simulink model "LoadFlow58BusNetwork_2023"  (R2023b)
settings: Solver=FixedStepDiscrete  StartTime=0.0  StopTime=4.5  FixedStep=75e-6  RelTol=1e-3  EnableMultiTasking=on
undefined symbols (not defined in the file): D1, D11, Delta
libraries: spsSeriesRLCBranchLib x41, spsLoadFlowBusLib x29, spsDistributedParametersLineLib x19, spsThreePhaseSeriesRLCLoadLib x15, spsThreePhaseTransformerTwoWindingsLib x13, spsThreePhaseParallelRLCLoadLib x11, spsThreePhaseVIMeasurementLib x11, spsSynchronousMachinepuStandardLib x7, spsExcitationSystemLib x7, spsHydraulicTurbineandGovernorLib x7, spsGenericPowerSystemStabilizerLib x7, spsMultiBandPowerSystemStabilizerLib x7
(part 1 of 5)
settings Model: Creator=The MathWorks, Inc.  LastModifiedBy=dilu2
settings SolverCC: AlgebraicLoopSolver=TrustRegion
settings DataIOCC: SaveFormat=StructureWithTime  SaveOutput=off  SignalLogging=off  DSMLogging=off  SaveTime=off  ReturnWorkspaceOutputs=off
settings OptimizationCC: ExpressionDepthLimit=2147483647  LifeSpan=inf
settings DebuggingCC: UnderspecifiedInitializationDetection=Classic  MergeDetectMultiDrivingBlocksExec=none  SolverPrmCheckMsg=warning  FcnCallInpInsideContextMsg=warning  UnconnectedInputMsg=warning  UnconnectedOutputMsg=warning  UnconnectedLineMsg=warning  StateNameClashWarn=warning  SFUnexpectedBacktrackingDiag=warning  SFNoUnconditionalDefaultTransitionDiag=warning  SFExecutionAtInitializationDiag=none  ArithmeticOperatorsInVariantConditions=warning
settings HardwareCC: ProdBitPerPointer=32  ProdBitPerSizeT=32  ProdBitPerPtrDiffT=32  ProdLargestAtomicFloat=None  ProdIntDivRoundTo=Undefined  ProdEndianess=Unspecified  ProdWordSize=32  ProdHWDeviceType=32-bit Generic
settings ModelReferenceCC: EnableRefExpFcnMdlSchedulingChecks=on  PropagateSignalLabelsOutOfModel=off
settings SFSimCC: SimUseLocalCustomCode=off  CustomCodeUndefinedFunction=UseInterfaceOnly
settings RTWCC: RTWUseLocalCustomCode=off
settings CodeAppCC: StateflowObjectComments=on
settings GRTTargetCC: TargetLangStandard=C89/C90 (ANSI)  CombineOutputUpdateFcns=off  GRTInterface=on
settings ConfigComp: CovMetricSettings=dw  CovSaveCumulativeToWorkspaceVar=on  CovSaveSingleToWorkspaceVar=on  CovExternalEMLEnable=off  CovSFcnEnable=off
settings SimscapeCC: SimscapeNormalizeSystem=off

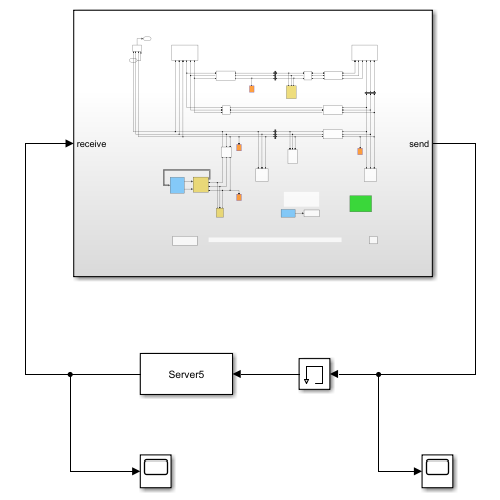
[thumbnail: Simulink's stored preview of the top-level diagram]
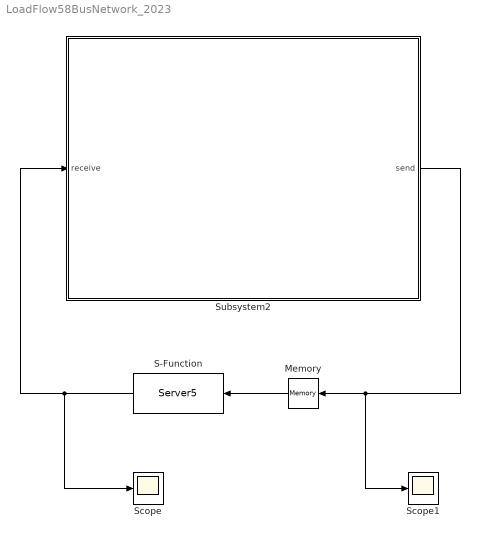
== system LoadFlow58BusNetwork_2023 ==
  Memory : Memory
  S-Function : S-Function  FunctionName=Server5  SFunctionDeploymentMode=off  EnableBusSupport=off
  Scope : Scope
  Scope1 : Scope
  Subsystem2 : Subsystem
  wires:
  Memory/1 -> S-Function/1
  Subsystem2/1(send) -> Scope1/1, Memory/1
  S-Function/1 -> Scope/1, Subsystem2/1(receive)

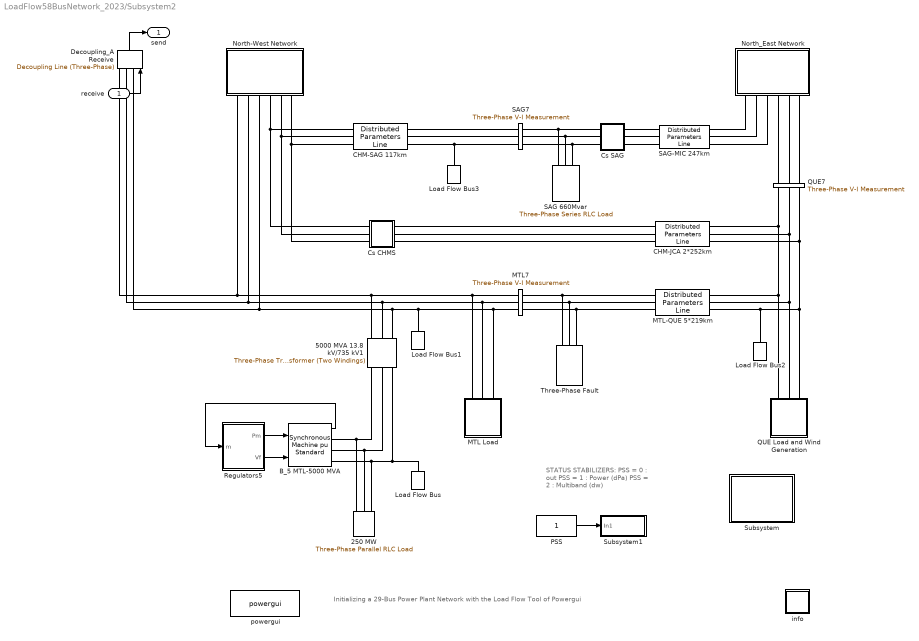
== system LoadFlow58BusNetwork_2023/Subsystem2 ==
  note: Initializing a 29-Bus Power Plant Network with the Load Flow Tool of Powergui
  note: STATUS STABILIZERS:
      | PSS = 0 :  out
      | PSS = 1 :  Power (dPa)
      | PSS = 2 :  Multiband (dw)
  receive : Inport
  250 MW : spsThreePhaseParallelRLCLoadLib/Three-Phase Parallel RLC Load  LConnTagsString=A|B|C  Configuration=Y (grounded)  NominalVoltage=(13800)*1  Vabc=[1e3 1e3 1e3]  Vabcp=[1e3 1e3 1e3]  NominalFrequency=60  UnbalancedPower=off  ActivePower=250000000  InductivePower=0  CapacitivePower=0  Pabc=[10e3 9e3 11e3]  QLabc=[100 90 110]  QCabc=[100 90 110]  Pabcp=[10e3 9e3 11e3]  QLabcp=[100 90 110]  QCabcp=[100 90 110]  Measurements=None  LoadType=constant PQ
  5000 MVA 13.8 kV/735 kV1 : spsThreePhaseTransformerTwoWindingsLib/Three-Phase Transformer (Two Windings)  Winding1Connection=Delta (D1)  Winding2Connection=Yg  CoreType=Three single-phase transformers  SetSaturation=off  Hysteresis=off  DataFile='basic_model'  SetInitialFlux=off  Measurements=None  UNITS=pu  NominalPower=[ 5000e6 60 ]  Winding1="[ 13.8e3 0.002  0.0]"  Winding2=[ 735e3 0.002 0.12]  Rm=500  Lm=500  L0=0.5  Saturation="[ 0,0  ;  0.005,1.2  ;  1.0,1.4 ]"  InitialFluxes=[ 0.8 , -0.8 , 0.7 ]  BreakLoop=off  DiscreteSolver=Trapezoidal iterative  DataType=off  TransfoNumber=0
  B_5 MTL-5000 MVA : spsSynchronousMachinepuStandardLib/Synchronous Machine pu Standard  PresetModel=No  MechanicalLoad=Mechanical power Pm  ShowDetailedParameters=on  RotorType=Salient-pole  Units=per unit standard parameters  MeasurementBus=off  NominalParameters="[5000E6  13800   60 ]"  Reactances1=[ 31 32 33 34 35 36 37 ]  Reactances2=[ 1.305, 0.296, 0.252, 0.474, 0.243, 0.18 ]  dAxisTimeConstants=Short-circuit  qAxisTimeConstants=Open-circuit  TimeConstants1=[]  TimeConstants2=[]  TimeConstants3=[]  TimeConstants4=[]  TimeConstants5=[ 1.01, 0.053, 0.1 ]  TimeConstants6=[]  TimeConstants7=[]  TimeConstants8=[]  StatorResistance=2.8544e-3  Mechanical="[ 3.7 0  32]"  PolePairs=32  InitialConditions=[0 -113.876 0.904539 0.904539 0.904539 -42.1129 -162.113 77.8871 1.28555]  SetSaturation=off  Saturation=[0.6404,0.7127,0.8441,0.9214,0.9956,1.082,1.19,1.316,1.457;0.7,0.7698,0.8872,0.9466,0.9969,1.046,1.1,1.151,1.201]  LoadFlowParameters=[1 4000000000 0 0 0]  TsPowergui=0  TsBlock=-1  IterativeModel=Trapezoidal non iterative  IterativeDiscreteModel=Trapezoidal non iterative  BusType=PV  Pref=4500000000  Qref=0  Qmin=-Inf  Qmax=Inf  PLF=0  QLF=0
  CHM-JCA 2*252km : spsDistributedParametersLineLib/Distributed Parameters Line  Phases=3  Length=252  Frequency=60  Resistance="[0.01273  0.3864]/2"  Inductance="[0.9337e-3  4.1264e-3]/2"  Capacitance=[12.74e-9 7.751e-9]*2  x1=[-0.0015 2.03674165345122e-08 15714.2625948716 -742648.807936692;-0.001425 2.03855691202494e-08 36703.0761534828 -741907.711972198;-0.00135 2.03874257939416e-08 57662.5498345927 -740573.546334321;-0.001275 2.03729850713921e-08 78575.9289556316 -738647.377534661;-0.0012 2.03422584962937e-08 99426.4956813152 -736130.745323082;-0.001125 2.02952706310004e-08 120197.582387628 -733025.661456871;-0.00105 2.02320590368927e-08 140872.584985664 -729334.60809256;-0.000975 2.01526742443518e-08 161434.976194686 -725060.535801733;-0.0009 2.00571797123662e-08 181868.318753776 -720206.861212384;-0.000825 1.99456517778037e-08 202156.278561532 -714777.464277717;-0.00075 1.98181795943887e-08 222282.637733301 -708776.685174569;-0.000675 1.96748650614343e-08 242231.307565505 -702209.320833938;-0.0006 1.95158227423853e-08 261986.341396704 -695080.621106396;-0.000525 1.93411797732382e-08 281531.947355116 -687396.284565432;-0.00045 1.91510757609102e-08 300852.500982395 -679162.453952101;-0.000375 1.89456626716403e-08 319932.557723587 -670385.711264616;-0.0003 1.87251047095091e-08 338756.865273267 -661073.072496791;-0.000225 1.84895781851768e-08 357310.375768001 -651231.982029569;-0.00015 1.82392713749432e-08 375578.257815379 -640870.306680096;-7.5e-05 1.79743843702428e-08 393545.908349999 -629996.329413108]  x2=[-0.0015 1.37869966912524e-08 -209700.60363331 -700128.672634898;-0.001425 1.37569590076229e-08 -189823.746323567 -705777.19657371;-0.00135 1.37159242214512e-08 -169795.146815414 -710861.533020335;-0.001275 1.36639251353176e-08 -149630.815664849 -715377.617634008;-0.0012 1.36010033164958e-08 -129346.87192967 -719321.84032579;-0.001125 1.35272090637252e-08 -108959.530284144 -722691.048144409;-0.00105 1.34426013670023e-08 -88485.0880572453 -725482.547796685;-0.000975 1.33472478604253e-08 -67939.9122048211 -727694.107800508;-0.0009 1.32412247681284e-08 -47340.4262260959 -729323.960268648;-0.000825 1.31246168433494e-08 -26703.0970349784 -730370.80232198;-0.00075 1.29975173006792e-08 -6044.42179666215 -730833.797130983;-0.000675 1.28600277415475e-08 14619.0852599556 -730712.574584693;-0.0006 1.27122580730043e-08 35270.906043496 -730007.231586556;-0.000525 1.25543264198615e-08 55894.5318044082 -728718.331976975;-0.00045 1.23863590302664e-08 76473.476331811 -726846.906082576;-0.000375 1.22084901747801e-08 96991.2891323175 -724394.449892584;-0.0003 1.20208620390443e-08 117431.568580308 -721362.923862956;-0.000225 1.18236246101198e-08 137777.975029139 -717754.751349214;-0.00015 1.16169355565895e-08 158014.243872805 -713572.81666926;-7.5e-05 1.14009601025203e-08 178124.198547619 -708820.46279769]  x3=[-0.0015 5.07994553465233e-11 0.894999888144781 -284.908126310178;-0.001425 5.0283598192617e-11 8.94952227203379 -284.768519995358;-0.00135 4.97275450996804e-11 16.9968905447508 -284.401274082759;-0.001275 4.91317405680481e-11 25.0306717632275 -283.806682143142;-0.0012 4.84966608747465e-11 33.0444438456788 -282.985219484209;-0.001125 4.78228136927654e-11 41.0318007053168 -281.937542770639;-0.00105 4.71107376852319e-11 48.9863573712786 -280.664489499167;-0.000975 4.63610020748113e-11 56.9017550926742 -279.1670773291;-0.0009 4.55742061886792e-11 64.7716664216747 -277.446503268816;-0.000825 4.47509789794286e-11 72.5898002715775 -275.504142718892;-0.00075 4.38919785222948e-11 80.3499069458043 -273.341548372634;-0.000675 4.29978914891001e-11 88.0457831338135 -270.960448974872;-0.0006 4.20694325993388e-11 95.6712768699312 -268.362747940034;-0.000525 4.11073440488415e-11 103.220292451139 -265.550521830581;-0.00045 4.0112394916475e-11 110.686795309884 -262.526018697035;-0.000375 3.90853805493524e-11 118.064816838024 -259.291656280926;-0.0003 3.80271219270451e-11 125.348459158035 -255.850020082081;-0.000225 3.69384650053039e-11 132.531899837691 -252.203861291819;-0.00015 3.58202800398148e-11 139.609396544424 -248.356094593689;-7.5e-05 3.46734608905305e-11 146.575291635653 -244.309795833516]  x4=[-0.0015 3.66725542612014e-11 -3172.83341993509 -10043.3125795462;-0.001425 3.78072265237595e-11 -2887.63550825212 -10128.9965094921;-0.00135 3.89116762679046e-11 -2600.12926492615 -10206.5834746072;-0.001275 3.99850206134097e-11 -2310.54451804911 -10276.0114530587;-0.0012 4.10264015452278e-11 -2019.11275723686 -10337.2249451828;-0.001125 4.20349865993756e-11 -1726.06694857993 -10390.1750178506;-0.00105 4.30099695283927e-11 -1431.64134841402 -10434.8193435841;-0.000975 4.39505709458435e-11 -1136.07131605904 -10471.1222343925;-0.0009 4.48560389493464e-11 -839.593125676469 -10499.0546703002;-0.000825 4.57256497216336e-11 -542.443777395441 -10518.5943225455;-0.00075 4.65587081091593e-11 -244.860807858432 -10529.7255714291;-0.000675 4.73545481777946e-11 52.9178996618857 -10532.4395188012;-0.0006 4.81125337451655e-11 350.654305422883 -10526.7339951737;-0.000525 4.88320588892069e-11 648.110403497316 -10512.6135614548;-0.00045 4.95125484325279e-11 945.048412031615 -10490.0895053033;-0.000375 5.01534584021993e-11 1241.23096332506 -10459.1798321051;-0.0003 5.07542764645976e-11 1536.4212935779 -10419.9092505798;-0.000225 5.13145223349566e-11 1830.38343215668 -10372.3091530296;-0.00015 5.18337481612995e-11 2122.8823902256 -10316.4175902441;-7.5e-05 5.23115388824452e-11 2413.68434859297 -10252.2792410835]  x5=0.00142516474882927  V1=ones(3,3)  V2=ones(3,3)  I1=ones(3,3)  I2=ones(3,3)  nHarmo=1  Measurements=None  Decoupling=on  VsMag0=[606505.937088283 606505.596193745 606505.952336163]  VrMag0=[596743.737336247 596743.91108333 596743.706580376]  VsAngle0=[3.61218308622859 -116.387796657598 123.612221103652]  VrAngle0=[-14.273856882172 -134.273869923449 105.726122150014]  IsMag0=[234.023435045969 234.01262310868 234.010085805348]  IrMag0=[8650.90032066037 8650.90619032997 8650.91364627855]  IsAngle0=[2.58186505622523 -117.420380634301 122.583034804805]  IrAngle0=[-15.1321830152103 -135.132103549667 104.867823050534]
      settings: AttributesFormatString=\n  LibrarySourceBlock=sps_lib/Power Grid Elements/Distributed Parameters Line
  CHM-SAG 117km : spsDistributedParametersLineLib/Distributed Parameters Line  Phases=3  Length=117  Frequency=60  Resistance="[0.01273  0.3864]"  Inductance="[0.9337e-3  4.1264e-3]"  Capacitance=[12.74e-9 7.751e-9]  x1=[-0.000675 1.89233254598605e-08 161384.253868475 -730188.013921104;-0.0006 1.87743600273455e-08 181962.578167373 -725333.731757204;-0.000525 1.86103866586821e-08 202395.444365406 -719899.628906115;-0.00045 1.84315364316721e-08 222666.518741967 -713890.049306513;-0.000375 1.82379523164507e-08 242759.596910358 -707309.796924379;-0.0003 1.80297890611975e-08 262658.616771325 -700164.131912787;-0.000225 1.78072130684338e-08 282347.671352857 -692458.766407013;-0.00015 1.75704022620027e-08 301811.021525973 -684199.859958349;-7.5e-05 1.73195459448395e-08 321033.108586345 -675394.014610243]  x2=[-0.000675 1.29805140179051e-08 211241.020698715 -709610.354234726;-0.0006 1.28522856813478e-08 231217.678579191 -703354.83438148;-0.000525 1.27137834242633e-08 251009.504585159 -696537.063435319;-0.00045 1.25651179632369e-08 270600.677433737 -689162.491418022;-0.000375 1.24064081391635e-08 289975.536241103 -681237.013449625;-0.0003 1.2237780822248e-08 309118.593041573 -672766.965035952;-0.000225 1.20593708105875e-08 328014.545168439 -663759.11700411;-0.00015 1.18713207224156e-08 346648.287486687 -654220.670089989;-7.5e-05 1.16737808820955e-08 365004.924467816 -644159.249182111]  x3=[-0.000675 1.55820323233606e-11 931.801693491444 -3923.77003572316;-0.0006 1.45506393837691e-11 1042.3568642954 -3895.85908672163;-0.000525 1.35076148856865e-11 1152.07879097064 -3864.83384757481;-0.00045 1.24537926069378e-11 1260.87976348777 -3830.71911938418;-0.000375 1.13900149569284e-11 1368.67280801408 -3793.54217294149;-0.0003 1.03171323032356e-11 1475.37175643905 -3753.33272692889;-0.000225 9.23600229183697e-12 1580.89131525588 -3710.12292416229;-0.00015 8.14748916152183e-12 1685.14713374373 -3663.94730589691;-7.5e-05 7.05246305303174e-12 1788.05587139649 -3614.84278421546]  x4=[-0.000675 2.73794343505806e-11 34.7429415929416 -1477.3234716751;-0.0006 2.81308416890378e-11 76.4934319413827 -1475.75088744227;-0.000525 2.88597616630651e-11 118.182774610719 -1472.99861052977;-0.00045 2.95656115851881e-11 159.777643778288 -1469.06884106565;-0.000375 3.0247827209779e-11 201.244789142101 -1463.96472044748;-0.0003 3.09058631841056e-11 242.551062500622 -1457.69032883121;-0.000225 3.15391934842784e-11 283.663444250935 -1450.25068186947;-0.00015 3.21473118357457e-11 324.549069784111 -1441.65172670223;-7.5e-05 3.27297321180019e-11 365.175255756669 -1431.90033720267]  x5=0.000661683633385019  V1=ones(3,3)  V2=ones(3,3)  I1=ones(3,3)  I2=ones(3,3)  nHarmo=1  Measurements=None  Decoupling=on  VsMag0=[610584.183721622 610584.009535668 610584.144430071]  VrMag0=[604521.569069031 604521.776249719 604521.565003274]  VsAngle0=[-2.95698942545205 -122.956984245963 117.043027319651]  VrAngle0=[1.15752648646157 -118.842485295537 121.157503589909]  IsMag0=[3301.92473587846 3301.92030404047 3301.91445622786]  IrMag0=[1209.87683704217 1209.8794095558 1209.88665322229]  IsAngle0=[-2.06102029188885 -122.06118186204 117.938965522645]  IrAngle0=[-14.0730509971519 -134.072584557023 105.927076719805]
      settings: AttributesFormatString=\n  LibrarySourceBlock=sps_lib/Power Grid Elements/Distributed Parameters Line
  Cs CHMS : Subsystem  mask{Xc=33/2}
      mask prompts: Xc "Condensator Reactance at  60Hz  (ohm):"
      mask help: Series Compensation
      mask init:
      | Cs=1/Xc/(2*pi*60);
      mask Display: disp('Cs')
  Cs SAG : Subsystem  mask{Xc=22}
      mask prompts: Xc "Condensator Reactance at  60Hz  (ohm):"
      mask help: Series Compensation
      mask init:
      | Cs=1/Xc/(2*pi*60);
      mask Display: disp('Cs')
  Decoupling_A Receive : spsDecouplingLineThreePhaseLib/Decoupling Line (Three-Phase)  Length=252  Frequency=60  Resistance="[0.01273  0.3864]/2"  Inductance="[0.9337e-3  4.1264e-3]/2"  Capacitance=[12.74e-9 7.751e-9]*2  VsMag0=[520613.013363981 520613.032750535 520613.04298088]  VsAngle0=[95.9069967092169 -144.093005822697 -24.0930027089988]  IhsMag0=[3886.83215054678 3886.83229528247 3886.83237166329]  IhsAngle0=[86.4922430478926 -153.507759484025 -33.5077563703669]  ShowPorts=on  ConnectorID=T34_3229_1960624034510_R
      settings: LibrarySourceBlock=|
      | sps_lib/Power Grid Elements/Decoupling Line
      | (Three-Phase)
  Load Flow Bus : spsLoadFlowBusLib/Load Flow Bus  LConnTagsString=a  Phases=single  Connectors=on one side  ID=MTL_13.8  Vbase=13.8e3  Vref=1  Vangle=0  VLF=1  VLFb=1  VLFc=1  angleLF=-47.86  angleLFb=0  angleLFc=0
      settings: AttributesFormatString=%<ID>\n%<Vbase>V\n%<VLF>pu\n%<angleLF>deg.
  Load Flow Bus1 : spsLoadFlowBusLib/Load Flow Bus  LConnTagsString=a  Phases=single  Connectors=on one side  ID=MTL7  Vbase=735e3  Vref=1  Vangle=0  VLF=1.013  VLFb=1  VLFc=1  angleLF=-23.64  angleLFb=0  angleLFc=0
      settings: AttributesFormatString=%<ID>\n%<Vbase>V\n%<VLF>pu\n%<angleLF>deg.
  Load Flow Bus2 : spsLoadFlowBusLib/Load Flow Bus  LConnTagsString=a  Phases=single  Connectors=on one side  ID=QUE7  Vbase=735e3  Vref=1  Vangle=0  VLF=1.023  VLFb=1  VLFc=1  angleLF=-14.99  angleLFb=0  angleLFc=0
      settings: AttributesFormatString=%<ID>\n%<Vbase>V\n%<VLF>pu\n%<angleLF>deg.
  Load Flow Bus3 : spsLoadFlowBusLib/Load Flow Bus  LConnTagsString=a  Phases=single  Connectors=on one side  ID=SAG7  Vbase=735e3  Vref=1  Vangle=0  VLF=1.036  VLFb=1  VLFc=1  angleLF=-0.1653  angleLFb=0  angleLFc=0
      settings: AttributesFormatString=%<ID>\n%<Vbase>V\n%<VLF>pu\n%<angleLF>deg.
  MTL Load : Subsystem
  MTL-QUE 5*219km : spsDistributedParametersLineLib/Distributed Parameters Line  Phases=3  Length=219  Frequency=60  Resistance="[0.01273  0.3864]/5"  Inductance="[0.9337e-3  4.1264e-3]/5"  Capacitance=[12.74e-9 7.751e-9]*5  x1=[-0.001275 8.55495292365405e-08 0 0;-0.0012 8.5539565073838e-08 0 0;-0.001125 8.54612218916147e-08 0 0;-0.00105 8.53145623162118e-08 0 0;-0.000975 8.50997035850499e-08 0 0;-0.0009 8.48168174529112e-08 0 0;-0.000825 8.44661300546415e-08 -143097.87967513 -713663.776535066;-0.00075 8.40479217243813e-08 -122864.998636675 -717423.987747196;-0.000675 8.35625267714708e-08 -102533.901198207 -720610.701200475;-0.0006 8.30103332132089e-08 -82120.839727942 -723221.369484929;-0.000525 8.23917824646769e-08 -61642.1321148898 -725253.905672274;-0.00045 8.17073689858793e-08 -41114.1487245812 -726706.684984182;-0.000375 8.0957639886479e-08 -20553.2993128498 -727578.546091098;-0.0003 8.01431944884468e-08 23.9800918763358 -727868.792040594;-0.000225 7.92646838469726e-08 20601.2403272839 -727577.190814499;-0.00015 7.83228102300215e-08 41162.0322463834 -726703.975514372;-7.5e-05 7.73183265569517e-08 61689.9198667053 -725249.844175161]  x2=[-0.001275 1.36639251353176e-08 0 0;-0.0012 1.36010033164958e-08 0 0;-0.001125 1.35272090637252e-08 0 0;-0.00105 1.34426013670023e-08 0 0;-0.000975 1.33472478604253e-08 0 0;-0.0009 1.32412247681284e-08 0 0;-0.000825 1.31246168433494e-08 -26703.0970349784 -730370.80232198;-0.00075 1.29975173006792e-08 -6044.42179666215 -730833.797130983;-0.000675 1.28600277415475e-08 14619.0852599556 -730712.574584693;-0.0006 1.27122580730043e-08 35270.906043496 -730007.231586556;-0.000525 1.25543264198615e-08 55894.5318044082 -728718.331976975;-0.00045 1.23863590302664e-08 76473.476331811 -726846.906082576;-0.000375 1.22084901747801e-08 96991.2891323175 -724394.449892584;-0.0003 1.20208620390443e-08 117431.568580308 -721362.923862956;-0.000225 1.18236246101198e-08 137777.975029139 -717754.751349214;-0.00015 1.16169355565895e-08 158014.243872805 -713572.81666926;-7.5e-05 1.14009601025203e-08 178124.198547619 -708820.46279769]  x3=[-0.001275 3.44514622141443e-10 0 0;-0.0012 3.20241684817421e-10 0 0;-0.001125 2.95712751190418e-10 0 0;-0.00105 2.70947429314669e-10 0 0;-0.000975 2.45965516209562e-10 0 0;-0.0009 2.20786982034195e-10 0 0;-0.000825 1.95431954123544e-10 -5323.24056616406 -20344.1866352289;-0.00075 1.69920700898976e-10 -4745.97060123277 -20486.5462812037;-0.000675 1.44273615665983e-10 -4164.90678001863 -20612.5292955361;-0.0006 1.18511200312087e-10 -3580.51359604976 -20722.0349693318;-0.000525 9.26540489179435e-11 -2993.2582042959 -20814.9757654308;-0.00045 6.67228312947496e-11 -2403.61004773192 -20891.2773883828;-0.000375 4.07382764611124e-11 -1812.04048207224 -20950.8788438377;-0.0003 1.47211560725886e-11 -1219.02239897635 -20993.7324873041;-0.000225 -1.13077321828583e-11 -625.029848026377 -21019.804062235;-0.00015 -3.73275812102124e-11 -30.5376577791733 -21029.0727274124;-7.5e-05 -6.33175911402782e-11 563.978943804418 -21021.531073607]  x4=[-0.001275 2.81063267851998e-10 0 0;-0.0012 3.09005352480878e-10 0 0;-0.001125 3.36700422958925e-10 0 0;-0.00105 3.64126340270548e-10 0 0;-0.000975 3.91261180557078e-10 0 0;-0.0009 4.18083252642368e-10 0 0;-0.000825 4.44571115372384e-10 -1592.00824148643 -5672.40977476447;-0.00075 4.70703594754937e-10 -1431.01007071873 -5715.14957068942;-0.000675 4.9645980088585e-10 -1268.86797239569 -5753.32076349229;-0.0006 5.21819144648024e-10 -1105.71156042984 -5786.89283970557;-0.000525 5.46761354170067e-10 -941.671259560544 -5815.83896232523;-0.00045 5.71266491031316e-10 -776.878201094405 -5840.13599226373;-0.000375 5.95314966200305e-10 -611.464118080948 -5859.76450684708;-0.0003 6.18887555693938e-10 -445.56124000721 -5874.70881534107;-0.000225 6.41965415944847e-10 -279.302187095527 -5884.95697149413;-0.00015 6.64530098864649e-10 -112.819864288947 -5890.50078308704;-7.5e-05 6.8656356659107e-10 53.7526449909449 -5891.33581848163]  x5=0.00123853603172068  V1=ones(3,3)  V2=ones(3,3)  I1=ones(3,3)  I2=ones(3,3)  nHarmo=1  Measurements=None  Decoupling=on  VsMag0=[594302.51828104 594302.525591461 594302.380387439]  VrMag0=[596743.737336247 596743.91108333 596743.706580376]  VsAngle0=[-23.5181046800016 -143.518120437638 96.4818868308225]  VrAngle0=[-14.273856882172 -134.273869923449 105.726122150014]  IsMag0=[17258.832188666 17258.8369567328 17258.8217052462]  IrMag0=[4835.28137561693 4835.27973459385 4835.28879561867]  IsAngle0=[-26.8431826212177 -146.843231946899 93.1567790076167]  IrAngle0=[-27.8572964469081 -147.85718369481 92.1427767692483]
      settings: AttributesFormatString=\n  LibrarySourceBlock=sps_lib/Power Grid Elements/Distributed Parameters Line
  MTL7 : spsThreePhaseVIMeasurementLib/Three-Phase V-I Measurement  VoltageMeasurement=phase-to-ground  SetLabelV=on  LabelV=Vabc_MTL7  Vpu=on  VpuLL=off  CurrentMeasurement=no  SetLabelI=off  LabelI=A1  Ipu=off  Pbase=100e6  Vbase=735e3  OutputType=Magnitude  PhasorSimulation=off  PSBequivalent=0
  North-West Network : Subsystem
  North_East Network : Subsystem
  PSS : Constant
  QUE Load and Wind Generation : Subsystem
  QUE7 : spsThreePhaseVIMeasurementLib/Three-Phase V-I Measurement  VoltageMeasurement=no  SetLabelV=on  LabelV=Vabc_QUE7  Vpu=on  VpuLL=off  CurrentMeasurement=no  SetLabelI=off  LabelI=A1  Ipu=off  Pbase=100e6  Vbase=735e3  OutputType=Magnitude  PhasorSimulation=off  PSBequivalent=0
  Regulators5 : Subsystem
  SAG 660Mvar : spsThreePhaseSeriesRLCLoadLib/Three-Phase Series RLC Load  LConnTagsString=A|B|C  Configuration=Y (grounded)  NominalVoltage=735e3  Vabc=[1e3 1e3 1e3]  Vabcp=[1e3 1e3 1e3]  NominalFrequency=60  UnbalancedPower=off  ActivePower=2200000  InductivePower=660e6  CapacitivePower=0  Pabc=[10e3 9e3 11e3]  QLabc=[100 90 110]  QCabc=[100 90 110]  Pabcp=[10e3 9e3 11e3]  QLabcp=[100 90 110]  QCabcp=[100 90 110]  Measurements=None  LoadType=constant Z
  SAG-MIC 247km : spsDistributedParametersLineLib/Distributed Parameters Line  Phases=3  Length=247  Frequency=60  Resistance="[0.01273  0.3864]/1"  Inductance="[0.9337e-3  4.1264e-3]/1"  Capacitance=[12.74e-9 7.751e-9]*1  x1=[-0.001425 1.43336889403955e-08 -23892.3616667391 -729222.084147031;-0.00135 1.43165005834428e-08 -3267.28940136649 -729606.070163574;-0.001275 1.42878678349735e-08 17360.3946851623 -729406.820250977;-0.0012 1.42478135835687e-08 37974.2011378027 -728624.493686569;-0.001125 1.4196369847984e-08 58557.6515950784 -727259.715850236;-0.00105 1.41335777515546e-08 79094.2919616311 -725313.5777245;-0.000975 1.40594874893215e-08 99567.7055613729 -722787.635022401;-0.0009 1.39741582879069e-08 119961.526260726 -719683.906943886;-0.000825 1.38776583581687e-08 140259.451551459 -716004.874561694;-0.00075 1.37700648406743e-08 160445.255582663 -711753.478838019;-0.000675 1.36514637440353e-08 180502.80213145 -706933.118273554;-0.0006 1.35219498761537e-08 200416.057501998 -701547.64619078;-0.000525 1.33816267684339e-08 220169.103342647 -695601.367653681;-0.00045 1.32306065930212e-08 239746.149370785 -689099.036026337;-0.000375 1.30690100731331e-08 259131.545995354 -682045.849173163;-0.0003 1.28969663865551e-08 278309.796826901 -674447.445303811;-0.000225 1.27146130623778e-08 297265.571065147 -666309.898466075;-0.00015 1.25220958710586e-08 315983.715754199 -657639.713690389;-7.5e-05 1.23195687078946e-08 334449.26789559 -648443.821789803]  x2=[-0.001425 4.57814854681873e-09 88893.3544414584 -739233.912944195;-0.00135 4.54232022260751e-09 109756.403307754 -736425.413361953;-0.001275 4.50286083711016e-09 130531.714584575 -733028.226571956;-0.0012 4.4598019335557e-09 151202.680805959 -729045.068233345;-0.001125 4.41317793257282e-09 171752.777917786 -724479.122421952;-0.00105 4.36302610467453e-09 192165.57848685 -719334.039084997;-0.000975 4.3093865404647e-09 212424.764832704 -713613.931123378;-0.0009 4.25230211859025e-09 232514.142071759 -707323.371103878;-0.000825 4.1918184714646e-09 252417.651063227 -700467.387603928;-0.00075 4.12798394878983e-09 272119.381246555 -693051.461191837;-0.000675 4.06084957890668e-09 291603.583360081 -685081.520045713;-0.0006 3.99046902800322e-09 310854.682030753 -676563.935214563;-0.000525 3.91689855721501e-09 329857.288224845 -667505.515525378;-0.00045 3.84019697765071e-09 348596.211549717 -657913.502140259;-0.000375 3.76042560337947e-09 367056.472396776 -647795.562767943;-0.0003 3.67764820241733e-09 385223.313915954 -637159.785534355;-0.000225 3.59193094575207e-09 403082.213812102 -626014.672517082;-0.00015 3.50334235444717e-09 420618.895953893 -614369.132948945;-7.5e-05 3.41195324486706e-09 437819.341785944 -602232.476096092]  x3=[-0.001425 1.37054247226365e-11 -591.222973545562 -3970.47337116299;-0.00135 1.31318183583394e-11 -478.7387494849 -3985.60043687573;-0.001275 1.25477146193703e-11 -365.871828992848 -3997.54147458096;-0.0012 1.19535804293209e-11 -252.712436158725 -4006.28693879584;-0.001125 1.13498907299722e-11 -139.351028869768 -4011.8298385301;-0.00105 1.07371281016331e-11 -25.8782265004741 -4014.16574287449;-0.000975 1.01157823773731e-11 87.6152625271343 -4013.29278454283;-0.0009 9.48635025145738e-12 201.038713254437 -4009.21166136463;-0.000825 8.84933488229663e-12 314.301456710359 -4001.92563572734;-0.00075 8.20524549023033e-12 427.312952390761 -3991.44053196837;-0.000675 7.55459695046361e-12 539.982860635129 -3977.76473171922;-0.0006 6.89790938148389e-12 652.221114842719 -3960.90916720538;-0.000525 6.23570772928618e-12 763.937993470423 -3940.88731250723;-0.00045 5.56852134773919e-12 875.044191754789 -3917.71517278904;-0.000375 4.89688357542806e-12 985.450893100892 -3891.41127150479;-0.0003 4.22133130931157e-12 1095.06984008095 -3861.99663559068;-0.000225 3.54240457553494e-12 1203.81340498599 -3829.49477865661;-0.00015 2.86064609774124e-12 1311.59465987403 -3793.93168218972;-7.5e-05 2.17660086322635e-12 1418.32744605905 -3755.33577478519]  x4=[-0.001425 1.02225474634085e-11 -44.2696955263392 -1445.03567527943;-0.00135 1.09039414844296e-11 -3.40032222025218 -1445.70991618334;-0.001275 1.15766190614639e-11 37.4717692513913 -1445.22847870036;-0.0012 1.22400424663487e-11 78.3139063640323 -1443.59174768424;-0.001125 1.28936813685648e-11 119.093440538169 -1440.80103151272;-0.00105 1.35370132591748e-11 159.77777323813 -1436.8585610416;-0.000975 1.41695238685088e-11 200.334382030847 -1431.76748782145;-0.0009 1.47907075772632e-11 240.730846583786 -1425.53188157832;-0.000825 1.54000678206857e-11 280.934874581273 -1418.15672696043;-0.00075 1.59971174855214e-11 320.914327538466 -1409.64791955353;-0.000675 1.65813792994032e-11 360.63724649238 -1400.01226116807;-0.0006 1.71523862123767e-11 400.071877549382 -1389.25745440194;-0.000525 1.77096817702523e-11 439.186697268776 -1377.39209648311;-0.00045 1.8252820479488e-11 477.950437862155 -1364.42567239717;-0.000375 1.87813681633099e-11 516.332112188395 -1350.36854730512;-0.0003 1.92949023087866e-11 554.301038524297 -1335.23195825768;-0.000225 1.97930124045796e-11 591.826865091093 -1319.02800521255;-0.00015 2.02753002690996e-11 628.87959431719 -1301.76964136186;-7.5e-05 2.0741380368807e-11 665.42960681777 -1283.4706627776]  x5=0.00139688767047948  V1=ones(3,3)  V2=ones(3,3)  I1=ones(3,3)  I2=ones(3,3)  nHarmo=1  Measurements=None  Decoupling=on  VsMag0=[595726.858585641 595726.856922628 595726.834929748]  VrMag0=[607930.231675994 607930.97680853 607930.152146888]  VsAngle0=[-1.09657636564441 -121.096578900449 118.90342250547]  VrAngle0=[7.63692875074741 -112.363120449619 127.636843332413]  IsMag0=[3296.72064632845 3296.71771518511 3296.71033953538]  IrMag0=[1187.28543067518 1187.29227239661 1187.29553954489]  IsAngle0=[-7.68926033426678 -127.689437762271 112.310695069133]  IrAngle0=[-0.975042579715418 -120.974669903303 119.024857828965]
      settings: AttributesFormatString=\n  LibrarySourceBlock=sps_lib/Power Grid Elements/Distributed Parameters Line
  SAG7 : spsThreePhaseVIMeasurementLib/Three-Phase V-I Measurement  VoltageMeasurement=no  SetLabelV=on  LabelV=Vabc_SAG7  Vpu=on  VpuLL=off  CurrentMeasurement=no  SetLabelI=off  LabelI=Iabc_SAG7  Ipu=off  Pbase=100e6  Vbase=735e3  OutputType=Magnitude  PhasorSimulation=off  PSBequivalent=0
  Subsystem : Subsystem
      mask Display: disp('Display\nWaveforms')
  Subsystem1 : Subsystem
      mask Display: disp('PSS_select')
  Three-Phase Fault : spsThreePhaseFaultLib/Three-Phase Fault  InitialStates=0  FaultA=on  FaultB=on  FaultC=on  GroundFault=on  SwitchTimes=[0.2 0.3]  External=off  SwitchStatus=NaN  FaultResistance=0.001  GroundResistance=0.001  SnubberResistance=1e6  SnubberCapacitance=inf  Measurements=None
  info : Subsystem
      settings: OpenFcn="showExample(\"simscapeelectricalsps/LoadFlow29BusNetworkExample\")"
      mask Display: disp('?')
  powergui : sps_lib/powergui  Priority=1  SimulationMode=Discrete  SampleTime=75e-6  frequency=60  Iterations=50  frequencyindice=60  Pbase=1e+008  ErrMax=0.0001  UnitsV=kV  UnitsW=MW  buscounter=0  FunctionMessages=off  echomessages=off  EnableUseOfTLC=off  CurrentSourceSwitches=off  DisableSnubberDevices=off  DisableRonSwitches=off  DisableVfSwitches=off  DisplayEquations=off  AutomaticDiscreteSolvers=off  SolverType=Tustin/Backward Euler (TBE)  Interpol=off  ExternalGateDelay=off  methode=off  Ts=100  x0status=blocks  SPID=off  SwTol=0  HookPort=off  NonlinearTolerance=1e-4  nMaxIteration=100  ContinueOnMaxIteration=off  RestoreLinks=warning  ResistiveCurrentMeasurement=off  Frange=[0:2:500]  Ylog=off  Xlog=on  ShowGrid=off  save=off  variable=ZData  structure=0  ZoomFFT=off  StartTime=0.0  cycles=1  DisplayStyle=1  fundamental=60  FreqAxis=off  MaxFrequency=1000  frequencyindicesteady=1  RmsSteady=1  display=off
  send : Outport
  wires:
  Regulators5/2(Vf) -> B_5 MTL-5000 MVA/2
  B_5 MTL-5000 MVA/1 -> Regulators5/1(m)
  receive/1 -> Decoupling_A Receive/1
  PSS/1 -> Subsystem1/1(In1)
  Regulators5/1(Pm) -> B_5 MTL-5000 MVA/1
  Decoupling_A Receive/1 -> send/1
  connections:
  SAG7/LConn1 -- CHM-SAG 117km/RConn1
  MTL7/RConn1 -- Three-Phase Fault/LConn1 -- MTL-QUE 5*219km/LConn1
  SAG-MIC 247km/RConn2 -- North_East Network/LConn2
  MTL7/RConn2 -- Three-Phase Fault/LConn2 -- MTL-QUE 5*219km/LConn2
  Load Flow Bus3/LConn1 -- SAG7/LConn3 -- CHM-SAG 117km/RConn3
  250 MW/LConn2 -- 5000 MVA 13.8 kV/735 kV1/LConn2 -- B_5 MTL-5000 MVA/RConn2
  Cs CHMS/LConn3 -- North-West Network/RConn6 -- CHM-SAG 117km/LConn3
  SAG-MIC 247km/RConn3 -- North_East Network/LConn3
  MTL7/LConn3 -- MTL Load/LConn3 -- Decoupling_A Receive/LConn1 -- North-West Network/RConn3 -- 5000 MVA 13.8 kV/735 kV1/RConn3 -- Load Flow Bus1/LConn1
  Cs SAG/RConn2 -- SAG-MIC 247km/LConn2
  Cs SAG/LConn2 -- SAG 660Mvar/LConn2 -- SAG7/RConn2
  5000 MVA 13.8 kV/735 kV1/LConn3 -- Load Flow Bus/LConn1 -- 250 MW/LConn3 -- B_5 MTL-5000 MVA/RConn3
  Cs SAG/LConn1 -- SAG 660Mvar/LConn1 -- SAG7/RConn1
  QUE Load and Wind Generation/LConn2 -- CHM-JCA 2*252km/RConn2 -- QUE7/LConn2 -- MTL-QUE 5*219km/RConn2
  Cs SAG/RConn1 -- SAG-MIC 247km/LConn1
  MTL7/LConn2 -- MTL Load/LConn2 -- Decoupling_A Receive/LConn2 -- North-West Network/RConn2 -- 5000 MVA 13.8 kV/735 kV1/RConn2
  QUE Load and Wind Generation/LConn1 -- CHM-JCA 2*252km/RConn1 -- QUE7/LConn1 -- MTL-QUE 5*219km/RConn1
  Cs CHMS/RConn2 -- CHM-JCA 2*252km/LConn2
  SAG7/LConn2 -- CHM-SAG 117km/RConn2
  Cs SAG/RConn3 -- SAG-MIC 247km/LConn3
  QUE7/RConn1 -- North_East Network/LConn4
  Cs SAG/LConn3 -- SAG 660Mvar/LConn3 -- SAG7/RConn3
  QUE7/RConn2 -- North_East Network/LConn5
  MTL7/LConn1 -- MTL Load/LConn1 -- Decoupling_A Receive/LConn3 -- North-West Network/RConn1 -- 5000 MVA 13.8 kV/735 kV1/RConn1
  QUE7/RConn3 -- North_East Network/LConn6
  MTL7/RConn3 -- Three-Phase Fault/LConn3 -- MTL-QUE 5*219km/LConn3
  SAG-MIC 247km/RConn1 -- North_East Network/LConn1
  QUE Load and Wind Generation/LConn3 -- CHM-JCA 2*252km/RConn3 -- QUE7/LConn3 -- MTL-QUE 5*219km/RConn3 -- Load Flow Bus2/LConn1
  Cs CHMS/LConn1 -- North-West Network/RConn4 -- CHM-SAG 117km/LConn1
  250 MW/LConn1 -- 5000 MVA 13.8 kV/735 kV1/LConn1 -- B_5 MTL-5000 MVA/RConn1
  Cs CHMS/LConn2 -- North-West Network/RConn5 -- CHM-SAG 117km/LConn2
  Cs CHMS/RConn3 -- CHM-JCA 2*252km/LConn3
  Cs CHMS/RConn1 -- CHM-JCA 2*252km/LConn1

== system LoadFlow58BusNetwork_2023/Subsystem2/Cs CHMS ==
  note: B
  Ca : spsSeriesRLCBranchLib/Series RLC Branch  LConnTagsString=__new0  RConnTagsString=__new0  BranchType=C  Resistance=1.0  Inductance=1.0  SetiL0=off  InitialCurrent=0  Capacitance=Cs  Setx0=off  InitialVoltage=0  Measurements=None
  Cb : spsSeriesRLCBranchLib/Series RLC Branch  LConnTagsString=__new0  RConnTagsString=__new0  BranchType=C  Resistance=1.0  Inductance=1.0  SetiL0=off  InitialCurrent=0  Capacitance=Cs  Setx0=off  InitialVoltage=0  Measurements=None
  Cc : spsSeriesRLCBranchLib/Series RLC Branch  LConnTagsString=__new0  RConnTagsString=__new0  BranchType=C  Resistance=1.0  Inductance=1.0  SetiL0=off  InitialCurrent=0  Capacitance=Cs  Setx0=off  InitialVoltage=0  Measurements=None
  A : PMIOPort  Side=Left
  B : PMIOPort  Port=2  Side=Left
  C : PMIOPort  Port=3  Side=Left
  "A " : PMIOPort  Port=4  Side=Right
  "B " : PMIOPort  Port=5  Side=Right
  "C " : PMIOPort  Port=6  Side=Right
  connections:
  Cc/RConn1 -- "C "/RConn1
  C/RConn1 -- Cc/LConn1
  Cb/RConn1 -- "B "/RConn1
  B/RConn1 -- Cb/LConn1
  Ca/RConn1 -- "A "/RConn1
  A/RConn1 -- Ca/LConn1

== system LoadFlow58BusNetwork_2023/Subsystem2/Cs SAG ==
  note: B
  Ca : spsSeriesRLCBranchLib/Series RLC Branch  LConnTagsString=__new0  RConnTagsString=__new0  BranchType=C  Resistance=1.0  Inductance=1.0  SetiL0=off  InitialCurrent=0  Capacitance=Cs  Setx0=off  InitialVoltage=0  Measurements=None
  Cb : spsSeriesRLCBranchLib/Series RLC Branch  LConnTagsString=__new0  RConnTagsString=__new0  BranchType=C  Resistance=1.0  Inductance=1.0  SetiL0=off  InitialCurrent=0  Capacitance=Cs  Setx0=off  InitialVoltage=0  Measurements=None
  Cc : spsSeriesRLCBranchLib/Series RLC Branch  LConnTagsString=__new0  RConnTagsString=__new0  BranchType=C  Resistance=1.0  Inductance=1.0  SetiL0=off  InitialCurrent=0  Capacitance=Cs  Setx0=off  InitialVoltage=0  Measurements=None
  A : PMIOPort  Side=Left
  B : PMIOPort  Port=2  Side=Left
  C : PMIOPort  Port=3  Side=Left
  "A " : PMIOPort  Port=4  Side=Right
  "B " : PMIOPort  Port=5  Side=Right
  "C " : PMIOPort  Port=6  Side=Right
  connections:
  A/RConn1 -- Ca/LConn1
  Ca/RConn1 -- "A "/RConn1
  B/RConn1 -- Cb/LConn1
  Cb/RConn1 -- "B "/RConn1
  C/RConn1 -- Cc/LConn1
  Cc/RConn1 -- "C "/RConn1

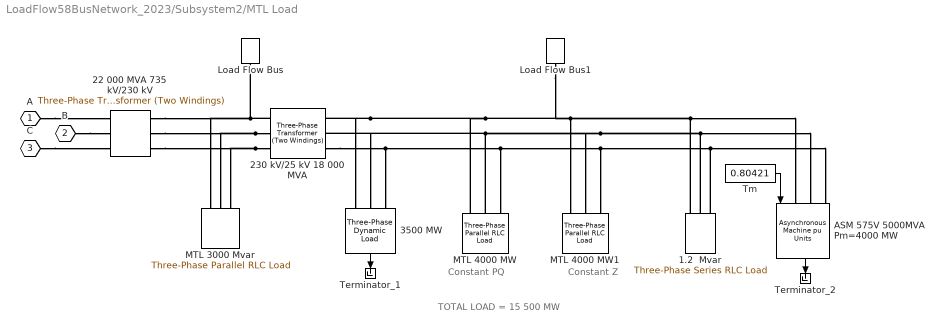
== system LoadFlow58BusNetwork_2023/Subsystem2/MTL Load ==
  note: Constant PQ
  note: Constant Z
  note: TOTAL LOAD = 15 500 MW
  1.2  Mvar : spsThreePhaseSeriesRLCLoadLib/Three-Phase Series RLC Load  LConnTagsString=A|B|C  Configuration=Y (grounded)  NominalVoltage=25e3  Vabc=[1e3 1e3 1e3]  Vabcp=[1e3 1e3 1e3]  NominalFrequency=60  UnbalancedPower=off  ActivePower=2000e6/50  InductivePower=0  CapacitivePower=2000e6  Pabc=[10e3 9e3 11e3]  QLabc=[100 90 110]  QCabc=[100 90 110]  Pabcp=[10e3 9e3 11e3]  QLabcp=[100 90 110]  QCabcp=[100 90 110]  Measurements=None  LoadType=constant Z
  22 000 MVA 735 kV/230 kV : spsThreePhaseTransformerTwoWindingsLib/Three-Phase Transformer (Two Windings)  Winding1Connection=Yg  Winding2Connection=Delta (D1)  CoreType=Three single-phase transformers  SetSaturation=off  Hysteresis=off  DataFile='basic_model'  SetInitialFlux=off  Measurements=None  UNITS=pu  NominalPower=[ 22000e6 60 ]  Winding1="[ 735e3 0.002  0.12]"  Winding2=[230e3 0.002 0]  Rm=500  Lm=500  L0=0.5  Saturation="[ 0,0  ;  0.005,1.2  ;  1.0,1.4 ]"  InitialFluxes=[ 0.8 , -0.8 , 0.7 ]  BreakLoop=off  DiscreteSolver=Trapezoidal iterative  DataType=off  TransfoNumber=0
  230 kV/25 kV 18 000 MVA : spsThreePhaseTransformerTwoWindingsLib/Three-Phase Transformer (Two Windings)  Winding1Connection=Yg  Winding2Connection=Delta (D1)  CoreType=Three single-phase transformers  SetSaturation=off  Hysteresis=off  DataFile='basic_model'  SetInitialFlux=off  Measurements=None  UNITS=pu  NominalPower=[18000e6 60 ]  Winding1="[ 230e3  0.08/30   0.08 ]"  Winding2="[ 25e3  0.08/30  0.08]"  Rm=500  Lm=500  L0=0.5  Saturation="[ 0,0  ;  0.005,1.2  ;  1.0,1.4 ]"  InitialFluxes=[ 0.8 , -0.8 , 0.7 ]  BreakLoop=off  DiscreteSolver=Trapezoidal iterative  DataType=off  TransfoNumber=0
  3500 MW : spsThreePhaseDynamicLoadLib/Three-Phase Dynamic Load  NominalVoltage=[ 25e3 60 ]  ActiveReactivePowers=[3.5e+09 4.44089e-08]  PositiveSequence=[0.991615 -96.3945]  ExternalControl=off  NpNq="[1.5  2.5]"  TimeConstants="[0  0  0  0]"  MinimumVoltage=0.7  Tfilter=1e-4  LoadFlowParameters=[4,0,0,0,0]
      settings: LibrarySourceBlock=|
      | sps_lib/Passives/Three-Phase
      | Dynamic Load
  ASM 575V 5000MVA Pm=4000 MW : spsAsynchronousMachinepuUnitsLib/Asynchronous Machine pu Units  RotorType=Squirrel-cage  PresetModel=No  MechanicalLoad=Torque Tm  ShowDetailedParameters=on  ReferenceFrame=Rotor  Units=pu  MeasurementBus=off  NominalParameters="[5000e6 25e3  60]"  VoltageRatio=1  Stator=[0.01117 0.04832]  Rotor=[0.006 0.04832]  Cage1=[0.01909 0.0397]  Cage2=[0.01909 0.0397]  Lm=2.424  Mechanical="[1  0   2]"  PolePairs=2  InitialConditions=[0.00523668 0 0.941796 0.941796 0.941796 -125.733 -245.733 -5.73298]  SimulateSaturation=off  Saturation="[0.212,0.4201,0.8125,1.0979,1.4799,2.2457,3.2586,4.5763,6.4763 ;   0.5,0.7,0.9,1,1.1,1.2 ,1.3,1.4,1.5]"  LoadFlowParameters=0  TsPowergui=0  TsBlock=-1  IterativeModel=Trapezoidal non iterative  IterativeDiscreteModel=Trapezoidal non iterative  Pmec=4000000000
      settings: LibrarySourceBlock=|
      | sps_lib/Electrical Machines/Asynchronous Machine
      | pu Units
  Load Flow Bus : spsLoadFlowBusLib/Load Flow Bus  LConnTagsString=a  Phases=single  Connectors=on one side  ID=MTL2  Vbase=230e3  Vref=1  Vangle=0  VLF=1.009  VLFb=1  VLFc=1  angleLF=-58.45  angleLFb=0  angleLFc=0
      settings: AttributesFormatString=%<ID>\n%<Vbase>V\n%<VLF>pu\n%<angleLF>deg.
  Load Flow Bus1 : spsLoadFlowBusLib/Load Flow Bus  LConnTagsString=a  Phases=single  Connectors=on one side  ID=MTL_25  Vbase=25e3  Vref=1  Vangle=0  VLF=0.9916  VLFb=1  VLFc=1  angleLF=-96.39  angleLFb=0  angleLFc=0
      settings: AttributesFormatString=%<ID>\n%<Vbase>V\n%<VLF>pu\n%<angleLF>deg.
  MTL 3000 Mvar : spsThreePhaseParallelRLCLoadLib/Three-Phase Parallel RLC Load  LConnTagsString=A|B|C  Configuration=Y (grounded)  NominalVoltage=230e3  Vabc=[1e3 1e3 1e3]  Vabcp=[1e3 1e3 1e3]  NominalFrequency=60  UnbalancedPower=off  ActivePower=0  InductivePower=0  CapacitivePower=3000e6  Pabc=[10e3 9e3 11e3]  QLabc=[100 90 110]  QCabc=[100 90 110]  Pabcp=[10e3 9e3 11e3]  QLabcp=[100 90 110]  QCabcp=[100 90 110]  Measurements=None  LoadType=constant Z
  MTL 4000 MW : spsThreePhaseParallelRLCLoadLib/Three-Phase Parallel RLC Load  LConnTagsString=A|B|C  Configuration=Y (grounded)  NominalVoltage=(25000)*0.991615  Vabc=[1e3 1e3 1e3]  Vabcp=[1e3 1e3 1e3]  NominalFrequency=60  UnbalancedPower=off  ActivePower=4000000000  InductivePower=0  CapacitivePower=0  Pabc=[10e3 9e3 11e3]  QLabc=[100 90 110]  QCabc=[100 90 110]  Pabcp=[10e3 9e3 11e3]  QLabcp=[100 90 110]  QCabcp=[100 90 110]  Measurements=None  LoadType=constant PQ
  MTL 4000 MW1 : spsThreePhaseParallelRLCLoadLib/Three-Phase Parallel RLC Load  LConnTagsString=A|B|C  Configuration=Y (grounded)  NominalVoltage=25e3  Vabc=[1e3 1e3 1e3]  Vabcp=[1e3 1e3 1e3]  NominalFrequency=60  UnbalancedPower=off  ActivePower=4000000000  InductivePower=0  CapacitivePower=0  Pabc=[10e3 9e3 11e3]  QLabc=[100 90 110]  QCabc=[100 90 110]  Pabcp=[10e3 9e3 11e3]  QLabcp=[100 90 110]  QCabcp=[100 90 110]  Measurements=None  LoadType=constant Z
  Terminator_1 : Terminator
  Terminator_2 : Terminator
  Tm : Constant  Value=0.80421
  A : PMIOPort  Side=Left
  B : PMIOPort  Port=2  Side=Left
  C : PMIOPort  Port=3  Side=Left
  wires:
  Tm/1 -> ASM 575V 5000MVA Pm=4000 MW/1
  3500 MW/1 -> Terminator_1/1
  ASM 575V 5000MVA Pm=4000 MW/1 -> Terminator_2/1
  connections:
  A/RConn1 -- 22 000 MVA 735 kV/230 kV/LConn1
  B/RConn1 -- 22 000 MVA 735 kV/230 kV/LConn2
  C/RConn1 -- 22 000 MVA 735 kV/230 kV/LConn3
  230 kV/25 kV 18 000 MVA/LConn1 -- Load Flow Bus/LConn1 -- 22 000 MVA 735 kV/230 kV/RConn1 -- MTL 3000 Mvar/LConn1
  230 kV/25 kV 18 000 MVA/LConn2 -- 22 000 MVA 735 kV/230 kV/RConn2 -- MTL 3000 Mvar/LConn2
  230 kV/25 kV 18 000 MVA/LConn3 -- 22 000 MVA 735 kV/230 kV/RConn3 -- MTL 3000 Mvar/LConn3
  MTL 4000 MW1/LConn1 -- Load Flow Bus1/LConn1 -- MTL 4000 MW/LConn1 -- 230 kV/25 kV 18 000 MVA/RConn1 -- 3500 MW/LConn1 -- ASM 575V 5000MVA Pm=4000 MW/LConn1 -- 1.2  Mvar/LConn1
  MTL 4000 MW1/LConn2 -- MTL 4000 MW/LConn2 -- 230 kV/25 kV 18 000 MVA/RConn2 -- 3500 MW/LConn2 -- ASM 575V 5000MVA Pm=4000 MW/LConn2 -- 1.2  Mvar/LConn2
  230 kV/25 kV 18 000 MVA/RConn3 -- ASM 575V 5000MVA Pm=4000 MW/LConn3 -- 1.2  Mvar/LConn3 -- MTL 4000 MW1/LConn3 -- MTL 4000 MW/LConn3 -- 3500 MW/LConn3
